simulink model "doppelpendelsim"  (Simulink 8.8)
settings: Solver=FixedStepAuto  StartTime=0.0  StopTime=10  FixedStep=0.0001  RelTol=1e-6  AbsTol=1e-6  EnableMultiTasking=on
undefined symbols (not defined in the file or in its folder): gdl, J1, J2, mdm, s1, s2
settings Model: Creator=ich  LastModifiedBy=ich  ExtModeTrigMode=oneshot  ExtModeArmWhenConnect=off
settings DataIOCC: LimitDataPoints=off  Refine=100
settings OptimizationCC: BlockReduction=off  BooleanDataType=off  InitFltsAndDblsToZero=on
settings DebuggingCC: SaveWithParameterizedLinksMsg=none  SignalResolutionControl=TryResolveAllWithWarning  MultiTaskDSMMsg=warning  MultiTaskCondExecSysMsg=none  StateNameClashWarn=none
settings HardwareCC: TargetUnknown=on
settings GRTTargetCC: TargetFcnLib=ansi_tfl_tmw.mat  ModelReferenceCompliant=off  GeneratePreprocessorConditionals=Use local settings  MatFileLogging=off

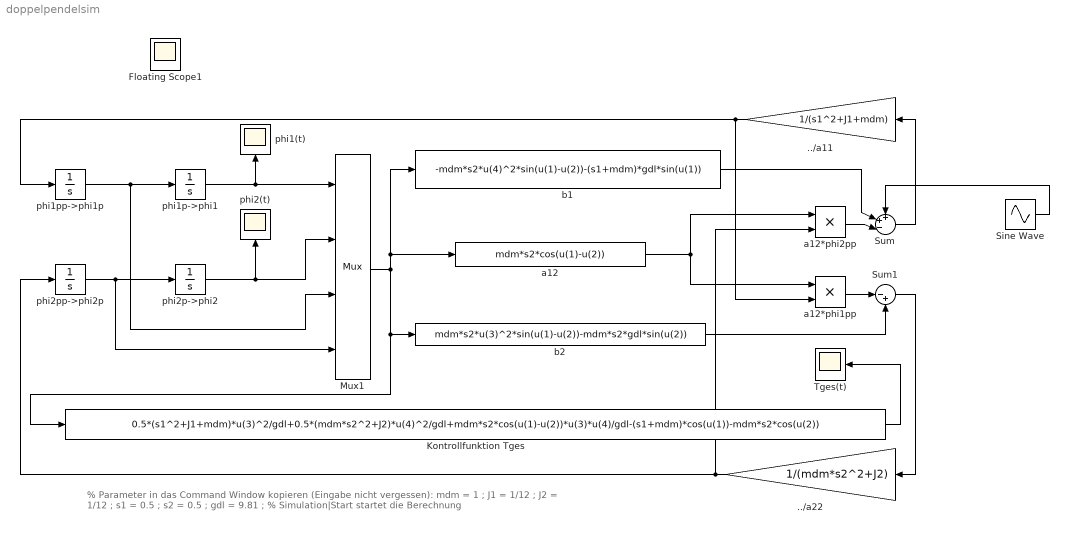
== system doppelpendelsim ==
  note: % Parameter in das Command Window kopieren (Eingabe nicht vergessen):
      | mdm = 1 ; J1 = 1/12 ; J2 = 1/12 ; s1 = 0.5 ; s2 = 0.5 ; gdl = 9.81 ;  % Simulation|Start startet die Berechnung
  ../a11 : Gain  Gain=1/(s1^2+J1+mdm)  SaturateOnIntegerOverflow=on  OutDataTypeStr=Inherit: Same as input  ParamDataTypeStr=Inherit: Same as input
  ../a22 : Gain  Gain=1/(mdm*s2^2+J2)  SaturateOnIntegerOverflow=on  OutDataTypeStr=Inherit: Same as input  ParamDataTypeStr=Inherit: Same as input
  Kontrollfunktion Tges : Fcn  Expr=0.5*(s1^2+J1+mdm)*u(3)^2/gdl+0.5*(mdm*s2^2+J2)*u(4)^2/gdl+mdm*s2*cos(u(1)-u(2))*u(3)*u(4)/gdl-(s1+mdm)*cos(u(1))-mdm*s2*cos(u(2))
  Mux1 : Mux
  Sine Wave : Sin  Amplitude=5  Frequency=2*pi*0.5  SampleTime=0
  Sum : Sum  Inputs=++-|  SaturateOnIntegerOverflow=on  InputSameDT=on  OutDataTypeStr=Inherit: Same as first input
  Sum1 : Sum  Inputs=|-+  SaturateOnIntegerOverflow=on  InputSameDT=on  OutDataTypeStr=Inherit: Same as first input
  Tges(t) : Scope
  a12 : Fcn  Expr=mdm*s2*cos(u(1)-u(2))
  a12*phi1pp : Product  SaturateOnIntegerOverflow=on  RndMeth=Zero  InputSameDT=on  OutDataTypeStr=Inherit: Same as first input
  a12*phi2pp : Product  SaturateOnIntegerOverflow=on  RndMeth=Zero  InputSameDT=on  OutDataTypeStr=Inherit: Same as first input
  b1 : Fcn  Expr=-mdm*s2*u(4)^2*sin(u(1)-u(2))-(s1+mdm)*gdl*sin(u(1))
  b2 : Fcn  Expr=mdm*s2*u(3)^2*sin(u(1)-u(2))-mdm*s2*gdl*sin(u(2))
  phi1(t) : Scope
  phi1p->phi1 : Integrator  InitialCondition=pi/2
  phi1pp->phi1p : Integrator
  phi2(t) : Scope
  phi2p->phi2 : Integrator
  phi2pp->phi2p : Integrator
  Floating Scope1 : Scope
  wires:
  phi2pp->phi2p/1 -> phi2p->phi2/1, Mux1/4
  a12*phi2pp/1 -> Sum/3
  Sum/1 -> ../a11/1
  a12*phi1pp/1 -> Sum1/1
  Sum1/1 -> ../a22/1
  Mux1/1 -> a12/1, b1/1, b2/1, Kontrollfunktion Tges/1
  a12/1 -> a12*phi2pp/1, a12*phi1pp/1
  b2/1 -> Sum1/2
  phi1p->phi1/1 -> phi1(t)/1, Mux1/1
  phi1pp->phi1p/1 -> phi1p->phi1/1, Mux1/3
  ../a11/1 -> phi1pp->phi1p/1, a12*phi1pp/2
  phi2p->phi2/1 -> Mux1/2, phi2(t)/1
  ../a22/1 -> phi2pp->phi2p/1, a12*phi2pp/2
  b1/1 -> Sum/2
  Kontrollfunktion Tges/1 -> Tges(t)/1
  Sine Wave/1 -> Sum/1
